simulink model "cppll"  (R2018a)
settings: Solver=VariableStepAuto  StartTime=0.0  StopTime=0.0003  MaxStep=2e-11  RelTol=1e-3
libraries: commsynccomp2 x2, dspswit3 x1, simulink_extras x1
Description:
  | Phase-Locked Loop (PLL)  Based Frequency Synthesis
  | 
  | This model shows how to simulate a phase-locked loop (PLL) frequency synthesizer.
settings Model: ExtModeAutoUpdateStatusClock=off  Creator=The MathWorks, Inc.  LastModifiedBy=肖
settings DataIOCC: LimitDataPoints=on  SaveFormat=Array
settings OptimizationCC: BlockReduction=off  BooleanDataType=off  LifeSpan=inf
settings DebuggingCC: SaveWithParameterizedLinksMsg=none  UnderspecifiedInitializationDetection=Classic  MergeDetectMultiDrivingBlocksExec=none  SignalResolutionControl=TryResolveAllWithWarning  SFUnexpectedBacktrackingDiag=warning  SFNoUnconditionalDefaultTransitionDiag=warning  SFExecutionAtInitializationDiag=none
settings HardwareCC: ProdBitPerPointer=32  ProdBitPerSizeT=32  ProdBitPerPtrDiffT=32  ProdLargestAtomicFloat=None  ProdIntDivRoundTo=Undefined  ProdEndianess=Unspecified  ProdWordSize=32  ProdHWDeviceType=32-bit Generic  TargetUnknown=on
settings ModelReferenceCC: PropagateSignalLabelsOutOfModel=off
settings CodeAppCC: StateflowObjectComments=on
settings GRTTargetCC: TargetLangStandard=C89/C90 (ANSI)  GeneratePreprocessorConditionals=Disable all
settings ConfigComp: CovMetricSettings=dw  CovHtmlReporting=on  CovSaveCumulativeToWorkspaceVar=on  CovSaveSingleToWorkspaceVar=on  CovExternalEMLEnable=off  CovSFcnEnable=off

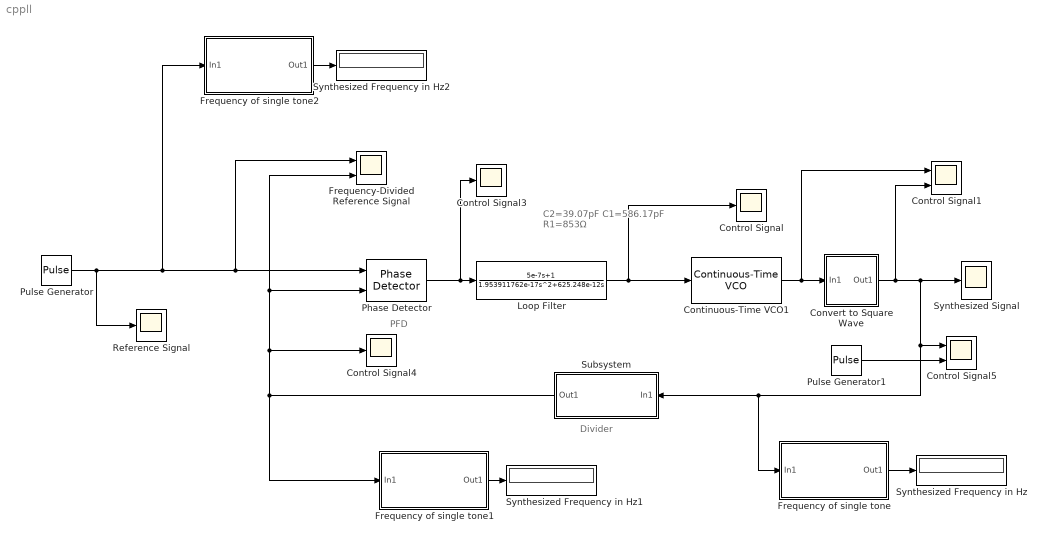
== system cppll ==
  note: PFD
  note: Divider
  note: C2=39.07pF
      | C1=586.17pF
      | R1=853Ω
  Continuous-Time VCO1 : commsynccomp2/Continuous-Time VCO  Ac=1  Fc=13.56e6  Kc=1000e6  Ph=0
      settings: SourceProductName=Communications System Toolbox  SourceProductBaseCode=CM
  Control Signal : Scope
  Control Signal1 : Scope  NumInputPorts=2
  Control Signal3 : Scope
  Control Signal4 : Scope
  Control Signal5 : Scope  NumInputPorts=2
  Convert to Square Wave : Subsystem
  Frequency of single tone : Subsystem
      mask Display: disp('Single Tone\nFrequency Estimator');
  Frequency of single tone1 : Subsystem
      mask Display: disp('Single Tone\nFrequency Estimator');
  Frequency of single tone2 : Subsystem
      mask Display: disp('Single Tone\nFrequency Estimator');
  Frequency-Divided Reference Signal : Scope  NumInputPorts=2
  Loop Filter : TransferFcn  Numerator=[5e-7, 1]  Denominator=[1.953911762e-17, 625.248e-12, 0]
  Phase Detector : commsynccomp2/Charge Pump PLL/Phase Detector  Thre=-sqrt(eps)  Cu=1e-5
      settings: SourceProductName=Communications System Toolbox  SourceProductBaseCode=CM
  Pulse Generator : DiscretePulseGenerator  PulseType=Time based  Period=1/(13.56e6)  PulseWidth=50
  Pulse Generator1 : DiscretePulseGenerator  PulseType=Time based  Period=1/(432e6)  PulseWidth=50
  Reference Signal : Scope
  Subsystem : Subsystem  Tag=Divider
      mask DialogControl Control2 Prompt: Divider
  Synthesized Signal : Scope
  Synthesized Frequency in Hz : Display
  Synthesized Frequency in Hz1 : Display
  Synthesized Frequency in Hz2 : Display
  wires:
  Continuous-Time VCO1/1 -> Control Signal1/1, Convert to Square Wave/1(In1)
  Frequency of single tone/1(Out1) -> Synthesized Frequency in Hz/1
  Frequency of single tone1/1(Out1) -> Synthesized Frequency in Hz1/1
  Phase Detector/1 -> Control Signal3/1, Loop Filter/1
  Loop Filter/1 -> Continuous-Time VCO1/1, Control Signal/1
  Pulse Generator/1 -> Frequency of single tone2/1(In1), Phase Detector/1, Frequency-Divided Reference Signal/1, Reference Signal/1
  Frequency of single tone2/1(Out1) -> Synthesized Frequency in Hz2/1
  Pulse Generator1/1 -> Control Signal5/2
  Subsystem/1(Out1) -> Frequency of single tone1/1(In1), Control Signal4/1, Frequency-Divided Reference Signal/2, Phase Detector/2
  Convert to Square Wave/1(Out1) -> Control Signal1/2, Subsystem/1(In1), Frequency of single tone/1(In1), Control Signal5/1, Synthesized Signal/1

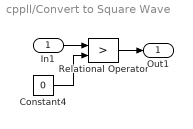
== system cppll/Convert to Square Wave ==
  In1 : Inport
  Constant4 : Constant  Value=0
  Relational Operator : RelationalOperator  Operator=>  RndMeth=Nearest  InputSameDT=on
  Out1 : Outport
  wires:
  Relational Operator/1 -> Out1/1
  In1/1 -> Relational Operator/1
  Constant4/1 -> Relational Operator/2

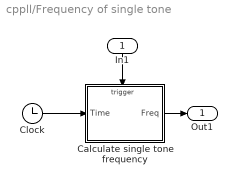
== system cppll/Frequency of single tone ==
  In1 : Inport
  Calculate single tone frequency : Subsystem  TreatAsAtomicUnit=on
  Clock : Clock
  Out1 : Outport
  wires:
  Calculate single tone frequency/1(Freq) -> Out1/1
  Clock/1 -> Calculate single tone frequency/1(Time)
  In1/1 -> Calculate single tone frequency/Trigger

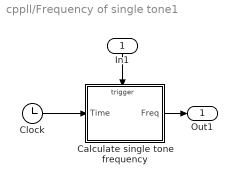
== system cppll/Frequency of single tone1 ==
  In1 : Inport
  Calculate single tone frequency : Subsystem  TreatAsAtomicUnit=on
  Clock : Clock
  Out1 : Outport
  wires:
  Calculate single tone frequency/1(Freq) -> Out1/1
  Clock/1 -> Calculate single tone frequency/1(Time)
  In1/1 -> Calculate single tone frequency/Trigger

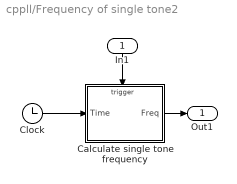
== system cppll/Frequency of single tone2 ==
  In1 : Inport
  Calculate single tone frequency : Subsystem  TreatAsAtomicUnit=on
  Clock : Clock
  Out1 : Outport
  wires:
  Calculate single tone frequency/1(Freq) -> Out1/1
  Clock/1 -> Calculate single tone frequency/1(Time)
  In1/1 -> Calculate single tone frequency/Trigger

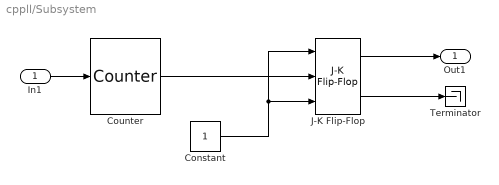
== system cppll/Subsystem ==
  In1 : Inport
  Constant : Constant
  Counter : dspswit3/Counter  Direction=Up  CountEvent=Either edge  CounterSize=User defined  MaxCount=32-1  InitialCount=0  Output=Hit  HitValue=32-1  ResetInput=off  SamplesPerFrame=1  Ts=1  CntDtype=double  HitDtype=Logical
  J-K Flip-Flop : simulink_extras/Flip Flops/J-K Flip-Flop  initial_condition=0
      settings: SourceProductName=Simulink
  Terminator : Terminator
  Out1 : Outport
  wires:
  In1/1 -> Counter/1
  J-K Flip-Flop/1 -> Out1/1
  J-K Flip-Flop/2 -> Terminator/1
  Counter/1 -> J-K Flip-Flop/2
  Constant/1 -> J-K Flip-Flop/3, J-K Flip-Flop/1

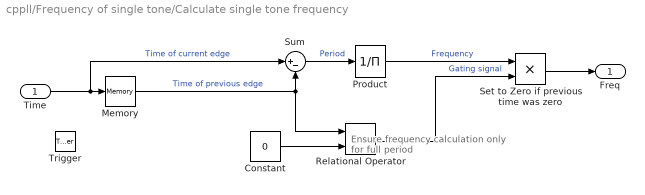
== system cppll/Frequency of single tone/Calculate single tone frequency ==
  note: Ensure frequency calculation
      | only for full period
  Time : Inport
  Trigger : TriggerPort  VariantControl=Variant  ZeroCross=off
  Constant : Constant  Value=0
  Memory : Memory  InheritSampleTime=on
  Product : Product  Inputs=/  SaturateOnIntegerOverflow=on  InputSameDT=on  OutDataTypeStr=Inherit: Same as first input
  Relational Operator : RelationalOperator  Operator=~=  RndMeth=Nearest  InputSameDT=on
  Set to Zero if previous time was zero : Product  SaturateOnIntegerOverflow=on  InputSameDT=on  OutDataTypeStr=Inherit: Same as first input
  Sum : Sum  Inputs=|+-  SaturateOnIntegerOverflow=on  InputSameDT=on  OutDataTypeStr=Inherit: Same as first input
  Freq : Outport  InitialOutput=0
  wires:
  Relational Operator/1 -> Set to Zero if previous time was zero/2  "Gating signal"
  Constant/1 -> Relational Operator/2
  Set to Zero if previous time was zero/1 -> Freq/1
  Memory/1 -> Relational Operator/1, Sum/2  "Time of previous edge"
  Product/1 -> Set to Zero if previous time was zero/1  "Frequency"
  Sum/1 -> Product/1  "Period"
  Time/1 -> Memory/1, Sum/1  "Time of current edge"

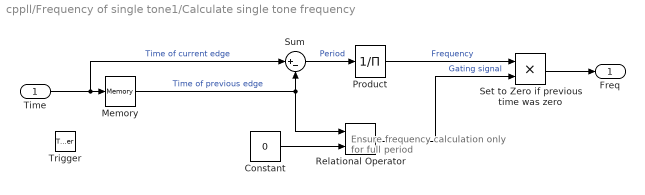
== system cppll/Frequency of single tone1/Calculate single tone frequency ==
  note: Ensure frequency calculation
      | only for full period
  Time : Inport
  Trigger : TriggerPort  VariantControl=Variant  ZeroCross=off
  Constant : Constant  Value=0
  Memory : Memory  InheritSampleTime=on
  Product : Product  Inputs=/  SaturateOnIntegerOverflow=on  InputSameDT=on  OutDataTypeStr=Inherit: Same as first input
  Relational Operator : RelationalOperator  Operator=~=  RndMeth=Nearest  InputSameDT=on
  Set to Zero if previous time was zero : Product  SaturateOnIntegerOverflow=on  InputSameDT=on  OutDataTypeStr=Inherit: Same as first input
  Sum : Sum  Inputs=|+-  SaturateOnIntegerOverflow=on  InputSameDT=on  OutDataTypeStr=Inherit: Same as first input
  Freq : Outport  InitialOutput=0
  wires:
  Relational Operator/1 -> Set to Zero if previous time was zero/2  "Gating signal"
  Constant/1 -> Relational Operator/2
  Set to Zero if previous time was zero/1 -> Freq/1
  Memory/1 -> Relational Operator/1, Sum/2  "Time of previous edge"
  Product/1 -> Set to Zero if previous time was zero/1  "Frequency"
  Sum/1 -> Product/1  "Period"
  Time/1 -> Memory/1, Sum/1  "Time of current edge"

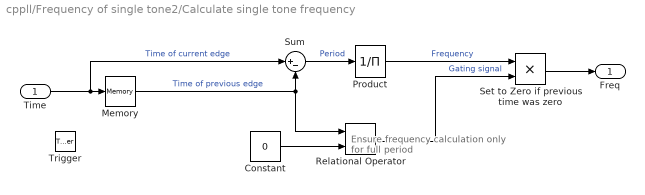
== system cppll/Frequency of single tone2/Calculate single tone frequency ==
  note: Ensure frequency calculation
      | only for full period
  Time : Inport
  Trigger : TriggerPort  VariantControl=Variant  ZeroCross=off
  Constant : Constant  Value=0
  Memory : Memory  InheritSampleTime=on
  Product : Product  Inputs=/  SaturateOnIntegerOverflow=on  InputSameDT=on  OutDataTypeStr=Inherit: Same as first input
  Relational Operator : RelationalOperator  Operator=~=  RndMeth=Nearest  InputSameDT=on
  Set to Zero if previous time was zero : Product  SaturateOnIntegerOverflow=on  InputSameDT=on  OutDataTypeStr=Inherit: Same as first input
  Sum : Sum  Inputs=|+-  SaturateOnIntegerOverflow=on  InputSameDT=on  OutDataTypeStr=Inherit: Same as first input
  Freq : Outport  InitialOutput=0
  wires:
  Relational Operator/1 -> Set to Zero if previous time was zero/2  "Gating signal"
  Constant/1 -> Relational Operator/2
  Set to Zero if previous time was zero/1 -> Freq/1
  Memory/1 -> Relational Operator/1, Sum/2  "Time of previous edge"
  Product/1 -> Set to Zero if previous time was zero/1  "Frequency"
  Sum/1 -> Product/1  "Period"
  Time/1 -> Memory/1, Sum/1  "Time of current edge"
